simulink model "designModel1"  (R2018b)
settings: Solver=VariableStepAuto  StartTime=0.0  StopTime=200  RelTol=1e-3
model workspace: external: MATLAB File C:\Users\Yavuz\Documents\MATLAB\constants.m (data not in the file)
libraries: cstblocks x1
settings Model: Creator=Yavuz  LastModifiedBy=Yavuz
settings DebuggingCC: AlgebraicLoopMsg=none

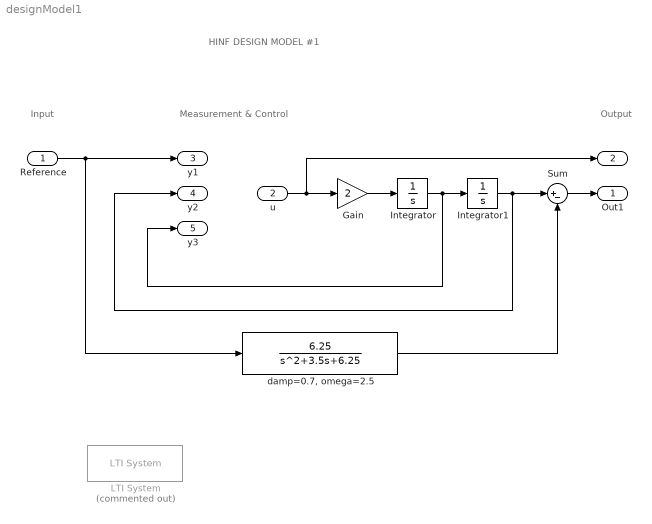
== system designModel1 ==
  note: Input
  note: Measurement & Control
  note: HINF DESIGN MODEL #1
  note: Output
  Reference : Inport
  u : Inport  Port=2
  Gain : Gain  Gain=2
  Integrator : Integrator
  Integrator1 : Integrator
  LTI System : cstblocks/LTI System  Commented=on  sys=K  IC=[]
  Sum : Sum  Inputs=|+-
  "damp=0.7, omega=2.5" : TransferFcn  Numerator=[6.25]  Denominator=[1 3.5 6.25]
  Out1 : Outport
  " " : Outport  Port=2
  y1 : Outport  Port=3
  y2 : Outport  Port=4
  y3 : Outport  Port=5
  wires:
  u/1 -> Gain/1, " "/1
  Integrator1/1 -> Sum/1, y2/1
  Reference/1 -> y1/1, "damp=0.7, omega=2.5"/1
  "damp=0.7, omega=2.5"/1 -> Sum/2
  Sum/1 -> Out1/1
  Gain/1 -> Integrator/1
  Integrator/1 -> Integrator1/1, y3/1
